simulink model "E55_1030"  (R2019b)
settings: Solver=FixedStepDiscrete  StartTime=0.0  StopTime=10  FixedStep=0.0005  RelTol=1e-3  EnableMultiTasking=on
InitFcn:
  | ecucoder_canfd
  | load('DATA_Plimit.mat')
  | a=0.775;
  | b=0.775;
  | kf=-50000;
  | kr=-50000;
  | m=226+75;
  | Iz=100;
  | u=0.85;
  | g=9.8;
  | L=a+b;
  | xi=0.1;
  | r=0.226;
  | Lw=1.171;
  | Tm=21;
  | i=15.9;
  | Jw=0.504;
  | Pmax=20000;
  | mw=19.3;
  | mb=148.9+75;
  | hg=0.280;
model workspace (MAT data in the model file):
  Initial_Steer_Position = 0
values from neighbouring files (symbols this model uses):
  SOC = [2.5 5 7.5 10 20 30 40 50 60 70 80 90 ... (14 elements, 14x1)]    [DATA_Plimit.mat]
  SOC_Discharge = [2.04592350211 2.57821618825 3.10671863859 3.63118835861 4.15200192786 4.66837694959 5.18149950051 5.69046162564 6.19532286188 6.696400261 7.19347596839 7.68712157998 ... (473 elements, 1x473)]    [DATA_Plimit.mat]
  VOLTAGE = [459.1488 476.0844 485.9448 487.344 492.822 498.8016 503.382 509.1108 518.8128 531.2472 544.5132 558.4656 ... (14 elements, 14x1)]    [DATA_Plimit.mat]
undefined symbols (not defined in the file or in its folder): DiscIntNeverNeededParam, H, HALL10, HALL6, HALL7, HALL8, HALL9, HPWM1, HPWM3, I_AN05_5V, I_AN07_5V, I_AN08_5V, I_AN09_5V, I_AN10_5V, I_SW11_H, I_SW12_H, I_SW13_H, I_SW14_H, I_SW15_H, I_SW16_H, I_SW17_H, I_SW18_H, I_SW19_H, LS1A2, O_HS1A2, O_HS1A8
libraries: ec311lib x152, simulink x92, canmsglib x30, canfdmsglib x2
(part 5 of 6)

== system E55_1030/Function-Call Subsystem2/Triggered Subsystem/AMK_Setpoints_Motor1 ==
  AMK_TorqueLimitNegativ_in : Inport
  AMK_TorqueLimitPositiv_in : Inport  Port=2
  AMK_TargetVelocity_in : Inport  Port=3
  AMK_Control_in : Inport  Port=4
  AMK_Control : Subsystem
  AMK_Setpoints_Motor1_DLC : Constant  Value=8  OutDataTypeStr=uint8
  AMK_Setpoints_Motor1_DLC_Out : Terminator
  AMK_Setpoints_Motor1_ID : Constant  Value=388  OutDataTypeStr=single
  AMK_Setpoints_Motor1_ID_Out : Terminator
  AMK_Setpoints_Motor1_mux : Mux  Inputs=8
  AMK_TargetVelocity : Subsystem
  AMK_TorqueLimitNegativ : Subsystem
  AMK_TorqueLimitPositiv : Subsystem
  Conv{1..8} (8 alike) : DataTypeConversion
  or{1..8} (8 alike) : simulink/Logic and Bit Operations/Bitwise Operator  logicop=OR  UseBitMask=off  NumInputPorts=4  BitMask=bin2dec('11011001')  BitMaskRealWorld=Stored Integer
  output : Outport
  wires:
  AMK_Setpoints_Motor1_mux/1 -> output/1
  AMK_TorqueLimitNegativ/1(output1) -> or1/1
  AMK_TorqueLimitNegativ/2(output2) -> or2/1
  AMK_TorqueLimitNegativ/3(output3) -> or3/1
  AMK_TorqueLimitNegativ/4(output4) -> or4/1
  AMK_TorqueLimitNegativ/5(output5) -> or5/1
  AMK_TorqueLimitNegativ/6(output6) -> or6/1
  AMK_TorqueLimitNegativ/7(output7) -> or7/1
  AMK_TorqueLimitNegativ/8(output8) -> or8/1
  AMK_TorqueLimitPositiv/1(output1) -> or1/2
  AMK_TorqueLimitPositiv/2(output2) -> or2/2
  AMK_TorqueLimitPositiv/3(output3) -> or3/2
  AMK_TorqueLimitPositiv/4(output4) -> or4/2
  AMK_TorqueLimitPositiv/5(output5) -> or5/2
  AMK_TorqueLimitPositiv/6(output6) -> or6/2
  AMK_TorqueLimitPositiv/7(output7) -> or7/2
  AMK_TorqueLimitPositiv/8(output8) -> or8/2
  AMK_TargetVelocity/1(output1) -> or1/3
  AMK_TargetVelocity/2(output2) -> or2/3
  AMK_TargetVelocity/3(output3) -> or3/3
  AMK_TargetVelocity/4(output4) -> or4/3
  AMK_TargetVelocity/5(output5) -> or5/3
  AMK_TargetVelocity/6(output6) -> or6/3
  AMK_TargetVelocity/7(output7) -> or7/3
  AMK_TargetVelocity/8(output8) -> or8/3
  AMK_Control/1(output1) -> or1/4
  AMK_Control/2(output2) -> or2/4
  AMK_Control/3(output3) -> or3/4
  AMK_Control/4(output4) -> or4/4
  AMK_Control/5(output5) -> or5/4
  AMK_Control/6(output6) -> or6/4
  AMK_Control/7(output7) -> or7/4
  AMK_Control/8(output8) -> or8/4
  or1/1 -> Conv1/1
  Conv1/1 -> AMK_Setpoints_Motor1_mux/1
  or2/1 -> Conv2/1
  Conv2/1 -> AMK_Setpoints_Motor1_mux/2
  or3/1 -> Conv3/1
  Conv3/1 -> AMK_Setpoints_Motor1_mux/3
  or4/1 -> Conv4/1
  Conv4/1 -> AMK_Setpoints_Motor1_mux/4
  or5/1 -> Conv5/1
  Conv5/1 -> AMK_Setpoints_Motor1_mux/5
  or6/1 -> Conv6/1
  Conv6/1 -> AMK_Setpoints_Motor1_mux/6
  or7/1 -> Conv7/1
  Conv7/1 -> AMK_Setpoints_Motor1_mux/7
  or8/1 -> Conv8/1
  Conv8/1 -> AMK_Setpoints_Motor1_mux/8
  AMK_Setpoints_Motor1_ID/1 -> AMK_Setpoints_Motor1_ID_Out/1
  AMK_Setpoints_Motor1_DLC/1 -> AMK_Setpoints_Motor1_DLC_Out/1
  AMK_TorqueLimitNegativ_in/1 -> AMK_TorqueLimitNegativ/1(AMK_TorqueLimitNegativ)
  AMK_TorqueLimitPositiv_in/1 -> AMK_TorqueLimitPositiv/1(AMK_TorqueLimitPositiv)
  AMK_TargetVelocity_in/1 -> AMK_TargetVelocity/1(AMK_TargetVelocity)
  AMK_Control_in/1 -> AMK_Control/1(AMK_Control)

== system E55_1030/Function-Call Subsystem2/Triggered Subsystem/AMK_Setpoints_Motor2 ==
  AMK_TorqueLimitNegativ_in : Inport
  AMK_TorqueLimitPositiv_in : Inport  Port=2
  AMK_TargetVelocity_in : Inport  Port=3
  AMK_Control_in : Inport  Port=4
  AMK_Control : Subsystem
  AMK_Setpoints_Motor1_DLC : Constant  Value=8  OutDataTypeStr=uint8
  AMK_Setpoints_Motor1_DLC_Out : Terminator
  AMK_Setpoints_Motor1_ID : Constant  Value=388  OutDataTypeStr=single
  AMK_Setpoints_Motor1_ID_Out : Terminator
  AMK_Setpoints_Motor1_mux : Mux  Inputs=8
  AMK_TargetVelocity : Subsystem
  AMK_TorqueLimitNegativ : Subsystem
  AMK_TorqueLimitPositiv : Subsystem
  Conv{1..8} (8 alike) : DataTypeConversion
  or{1..8} (8 alike) : simulink/Logic and Bit Operations/Bitwise Operator  logicop=OR  UseBitMask=off  NumInputPorts=4  BitMask=bin2dec('11011001')  BitMaskRealWorld=Stored Integer
  output : Outport
  wires:
  AMK_Control_in/1 -> AMK_Control/1(AMK_Control)
  AMK_TargetVelocity_in/1 -> AMK_TargetVelocity/1(AMK_TargetVelocity)
  AMK_TorqueLimitPositiv_in/1 -> AMK_TorqueLimitPositiv/1(AMK_TorqueLimitPositiv)
  AMK_TorqueLimitNegativ_in/1 -> AMK_TorqueLimitNegativ/1(AMK_TorqueLimitNegativ)
  AMK_Setpoints_Motor1_DLC/1 -> AMK_Setpoints_Motor1_DLC_Out/1
  AMK_Setpoints_Motor1_ID/1 -> AMK_Setpoints_Motor1_ID_Out/1
  Conv8/1 -> AMK_Setpoints_Motor1_mux/8
  or8/1 -> Conv8/1
  Conv7/1 -> AMK_Setpoints_Motor1_mux/7
  or7/1 -> Conv7/1
  Conv6/1 -> AMK_Setpoints_Motor1_mux/6
  or6/1 -> Conv6/1
  Conv5/1 -> AMK_Setpoints_Motor1_mux/5
  or5/1 -> Conv5/1
  Conv4/1 -> AMK_Setpoints_Motor1_mux/4
  or4/1 -> Conv4/1
  Conv3/1 -> AMK_Setpoints_Motor1_mux/3
  or3/1 -> Conv3/1
  Conv2/1 -> AMK_Setpoints_Motor1_mux/2
  or2/1 -> Conv2/1
  Conv1/1 -> AMK_Setpoints_Motor1_mux/1
  or1/1 -> Conv1/1
  AMK_Control/8(output8) -> or8/4
  AMK_Control/7(output7) -> or7/4
  AMK_Control/6(output6) -> or6/4
  AMK_Control/5(output5) -> or5/4
  AMK_Control/4(output4) -> or4/4
  AMK_Control/3(output3) -> or3/4
  AMK_Control/2(output2) -> or2/4
  AMK_Control/1(output1) -> or1/4
  AMK_TargetVelocity/8(output8) -> or8/3
  AMK_TargetVelocity/7(output7) -> or7/3
  AMK_TargetVelocity/6(output6) -> or6/3
  AMK_TargetVelocity/5(output5) -> or5/3
  AMK_TargetVelocity/4(output4) -> or4/3
  AMK_TargetVelocity/3(output3) -> or3/3
  AMK_TargetVelocity/2(output2) -> or2/3
  AMK_TargetVelocity/1(output1) -> or1/3
  AMK_TorqueLimitPositiv/8(output8) -> or8/2
  AMK_TorqueLimitPositiv/7(output7) -> or7/2
  AMK_TorqueLimitPositiv/6(output6) -> or6/2
  AMK_TorqueLimitPositiv/5(output5) -> or5/2
  AMK_TorqueLimitPositiv/4(output4) -> or4/2
  AMK_TorqueLimitPositiv/3(output3) -> or3/2
  AMK_TorqueLimitPositiv/2(output2) -> or2/2
  AMK_TorqueLimitPositiv/1(output1) -> or1/2
  AMK_TorqueLimitNegativ/8(output8) -> or8/1
  AMK_TorqueLimitNegativ/7(output7) -> or7/1
  AMK_TorqueLimitNegativ/6(output6) -> or6/1
  AMK_TorqueLimitNegativ/5(output5) -> or5/1
  AMK_TorqueLimitNegativ/4(output4) -> or4/1
  AMK_TorqueLimitNegativ/3(output3) -> or3/1
  AMK_TorqueLimitNegativ/2(output2) -> or2/1
  AMK_TorqueLimitNegativ/1(output1) -> or1/1
  AMK_Setpoints_Motor1_mux/1 -> output/1

== system E55_1030/Function-Call Subsystem2/Triggered Subsystem/AMK_Setpoints_Motor3 ==
  AMK_TorqueLimitNegativ_in : Inport
  AMK_TorqueLimitPositiv_in : Inport  Port=2
  AMK_TargetVelocity_in : Inport  Port=3
  AMK_Control_in : Inport  Port=4
  AMK_Control : Subsystem
  AMK_Setpoints_Motor1_DLC : Constant  Value=8  OutDataTypeStr=uint8
  AMK_Setpoints_Motor1_DLC_Out : Terminator
  AMK_Setpoints_Motor1_ID : Constant  Value=388  OutDataTypeStr=single
  AMK_Setpoints_Motor1_ID_Out : Terminator
  AMK_Setpoints_Motor1_mux : Mux  Inputs=8
  AMK_TargetVelocity : Subsystem
  AMK_TorqueLimitNegativ : Subsystem
  AMK_TorqueLimitPositiv : Subsystem
  Conv{1..8} (8 alike) : DataTypeConversion
  or{1..8} (8 alike) : simulink/Logic and Bit Operations/Bitwise Operator  logicop=OR  UseBitMask=off  NumInputPorts=4  BitMask=bin2dec('11011001')  BitMaskRealWorld=Stored Integer
  output : Outport
  wires:
  AMK_Control_in/1 -> AMK_Control/1(AMK_Control)
  AMK_TargetVelocity_in/1 -> AMK_TargetVelocity/1(AMK_TargetVelocity)
  AMK_TorqueLimitPositiv_in/1 -> AMK_TorqueLimitPositiv/1(AMK_TorqueLimitPositiv)
  AMK_TorqueLimitNegativ_in/1 -> AMK_TorqueLimitNegativ/1(AMK_TorqueLimitNegativ)
  AMK_Setpoints_Motor1_DLC/1 -> AMK_Setpoints_Motor1_DLC_Out/1
  AMK_Setpoints_Motor1_ID/1 -> AMK_Setpoints_Motor1_ID_Out/1
  Conv8/1 -> AMK_Setpoints_Motor1_mux/8
  or8/1 -> Conv8/1
  Conv7/1 -> AMK_Setpoints_Motor1_mux/7
  or7/1 -> Conv7/1
  Conv6/1 -> AMK_Setpoints_Motor1_mux/6
  or6/1 -> Conv6/1
  Conv5/1 -> AMK_Setpoints_Motor1_mux/5
  or5/1 -> Conv5/1
  Conv4/1 -> AMK_Setpoints_Motor1_mux/4
  or4/1 -> Conv4/1
  Conv3/1 -> AMK_Setpoints_Motor1_mux/3
  or3/1 -> Conv3/1
  Conv2/1 -> AMK_Setpoints_Motor1_mux/2
  or2/1 -> Conv2/1
  Conv1/1 -> AMK_Setpoints_Motor1_mux/1
  or1/1 -> Conv1/1
  AMK_Control/8(output8) -> or8/4
  AMK_Control/7(output7) -> or7/4
  AMK_Control/6(output6) -> or6/4
  AMK_Control/5(output5) -> or5/4
  AMK_Control/4(output4) -> or4/4
  AMK_Control/3(output3) -> or3/4
  AMK_Control/2(output2) -> or2/4
  AMK_Control/1(output1) -> or1/4
  AMK_TargetVelocity/8(output8) -> or8/3
  AMK_TargetVelocity/7(output7) -> or7/3
  AMK_TargetVelocity/6(output6) -> or6/3
  AMK_TargetVelocity/5(output5) -> or5/3
  AMK_TargetVelocity/4(output4) -> or4/3
  AMK_TargetVelocity/3(output3) -> or3/3
  AMK_TargetVelocity/2(output2) -> or2/3
  AMK_TargetVelocity/1(output1) -> or1/3
  AMK_TorqueLimitPositiv/8(output8) -> or8/2
  AMK_TorqueLimitPositiv/7(output7) -> or7/2
  AMK_TorqueLimitPositiv/6(output6) -> or6/2
  AMK_TorqueLimitPositiv/5(output5) -> or5/2
  AMK_TorqueLimitPositiv/4(output4) -> or4/2
  AMK_TorqueLimitPositiv/3(output3) -> or3/2
  AMK_TorqueLimitPositiv/2(output2) -> or2/2
  AMK_TorqueLimitPositiv/1(output1) -> or1/2
  AMK_TorqueLimitNegativ/8(output8) -> or8/1
  AMK_TorqueLimitNegativ/7(output7) -> or7/1
  AMK_TorqueLimitNegativ/6(output6) -> or6/1
  AMK_TorqueLimitNegativ/5(output5) -> or5/1
  AMK_TorqueLimitNegativ/4(output4) -> or4/1
  AMK_TorqueLimitNegativ/3(output3) -> or3/1
  AMK_TorqueLimitNegativ/2(output2) -> or2/1
  AMK_TorqueLimitNegativ/1(output1) -> or1/1
  AMK_Setpoints_Motor1_mux/1 -> output/1

== system E55_1030/Function-Call Subsystem2/Triggered Subsystem/AMK_Setpoints_Motor4 ==
  AMK_TorqueLimitNegativ_in : Inport
  AMK_TorqueLimitPositiv_in : Inport  Port=2
  AMK_TargetVelocity_in : Inport  Port=3
  AMK_Control_in : Inport  Port=4
  AMK_Control : Subsystem
  AMK_Setpoints_Motor1_DLC : Constant  Value=8  OutDataTypeStr=uint8
  AMK_Setpoints_Motor1_DLC_Out : Terminator
  AMK_Setpoints_Motor1_ID : Constant  Value=388  OutDataTypeStr=single
  AMK_Setpoints_Motor1_ID_Out : Terminator
  AMK_Setpoints_Motor1_mux : Mux  Inputs=8
  AMK_TargetVelocity : Subsystem
  AMK_TorqueLimitNegativ : Subsystem
  AMK_TorqueLimitPositiv : Subsystem
  Conv{1..8} (8 alike) : DataTypeConversion
  or{1..8} (8 alike) : simulink/Logic and Bit Operations/Bitwise Operator  logicop=OR  UseBitMask=off  NumInputPorts=4  BitMask=bin2dec('11011001')  BitMaskRealWorld=Stored Integer
  output : Outport
  wires:
  AMK_Setpoints_Motor1_mux/1 -> output/1
  AMK_TorqueLimitNegativ/1(output1) -> or1/1
  AMK_TorqueLimitNegativ/2(output2) -> or2/1
  AMK_TorqueLimitNegativ/3(output3) -> or3/1
  AMK_TorqueLimitNegativ/4(output4) -> or4/1
  AMK_TorqueLimitNegativ/5(output5) -> or5/1
  AMK_TorqueLimitNegativ/6(output6) -> or6/1
  AMK_TorqueLimitNegativ/7(output7) -> or7/1
  AMK_TorqueLimitNegativ/8(output8) -> or8/1
  AMK_TorqueLimitPositiv/1(output1) -> or1/2
  AMK_TorqueLimitPositiv/2(output2) -> or2/2
  AMK_TorqueLimitPositiv/3(output3) -> or3/2
  AMK_TorqueLimitPositiv/4(output4) -> or4/2
  AMK_TorqueLimitPositiv/5(output5) -> or5/2
  AMK_TorqueLimitPositiv/6(output6) -> or6/2
  AMK_TorqueLimitPositiv/7(output7) -> or7/2
  AMK_TorqueLimitPositiv/8(output8) -> or8/2
  AMK_TargetVelocity/1(output1) -> or1/3
  AMK_TargetVelocity/2(output2) -> or2/3
  AMK_TargetVelocity/3(output3) -> or3/3
  AMK_TargetVelocity/4(output4) -> or4/3
  AMK_TargetVelocity/5(output5) -> or5/3
  AMK_TargetVelocity/6(output6) -> or6/3
  AMK_TargetVelocity/7(output7) -> or7/3
  AMK_TargetVelocity/8(output8) -> or8/3
  AMK_Control/1(output1) -> or1/4
  AMK_Control/2(output2) -> or2/4
  AMK_Control/3(output3) -> or3/4
  AMK_Control/4(output4) -> or4/4
  AMK_Control/5(output5) -> or5/4
  AMK_Control/6(output6) -> or6/4
  AMK_Control/7(output7) -> or7/4
  AMK_Control/8(output8) -> or8/4
  or1/1 -> Conv1/1
  Conv1/1 -> AMK_Setpoints_Motor1_mux/1
  or2/1 -> Conv2/1
  Conv2/1 -> AMK_Setpoints_Motor1_mux/2
  or3/1 -> Conv3/1
  Conv3/1 -> AMK_Setpoints_Motor1_mux/3
  or4/1 -> Conv4/1
  Conv4/1 -> AMK_Setpoints_Motor1_mux/4
  or5/1 -> Conv5/1
  Conv5/1 -> AMK_Setpoints_Motor1_mux/5
  or6/1 -> Conv6/1
  Conv6/1 -> AMK_Setpoints_Motor1_mux/6
  or7/1 -> Conv7/1
  Conv7/1 -> AMK_Setpoints_Motor1_mux/7
  or8/1 -> Conv8/1
  Conv8/1 -> AMK_Setpoints_Motor1_mux/8
  AMK_Setpoints_Motor1_ID/1 -> AMK_Setpoints_Motor1_ID_Out/1
  AMK_Setpoints_Motor1_DLC/1 -> AMK_Setpoints_Motor1_DLC_Out/1
  AMK_TorqueLimitNegativ_in/1 -> AMK_TorqueLimitNegativ/1(AMK_TorqueLimitNegativ)
  AMK_TorqueLimitPositiv_in/1 -> AMK_TorqueLimitPositiv/1(AMK_TorqueLimitPositiv)
  AMK_TargetVelocity_in/1 -> AMK_TargetVelocity/1(AMK_TargetVelocity)
  AMK_Control_in/1 -> AMK_Control/1(AMK_Control)

== system E55_1030/Function-Call Subsystem2/计算理想横摆角速度和质心侧偏角/线性二自由度模型 ==
  steer_angle_rad : Inport
  velocity_m/s : Inport  Port=2
  Add : Sum  Inputs=++-
  Add1 : Sum  Inputs=+-
  Add2 : Sum  Inputs=++-
  Discrete-Time Integrator : DiscreteIntegrator  SampleTime=-1  ICPrevOutput=DiscIntNeverNeededParam  ICPrevScaledInput=DiscIntNeverNeededParam
  Discrete-Time Integrator1 : DiscreteIntegrator  SampleTime=-1  ICPrevOutput=DiscIntNeverNeededParam  ICPrevScaledInput=DiscIntNeverNeededParam
  Divide{,1..2,4} (4 alike) : Product  Inputs=*/
  Divide3 : Product  Inputs=**
  Gain2 : Gain  Gain=kf+kr
  Gain3 : Gain  Gain=a*kf-b*kr
  Gain4 : Gain  Gain=kf
  Gain5 : Gain  Gain=a*kf-b*kr
  Gain6 : Gain  Gain=a^2*kf+b^2*kr
  Gain7 : Gain  Gain=a*kr
  Gain8 : Gain  Gain=180/pi
  Gain9 : Gain  Gain=180/pi
  Iz_kg*m^2 : Constant  Value=Iz
  m_kg : Constant  Value=m
  side_slip_angle_° : Outport
  yaw_rate_°/s : Outport  Port=2
  wires:
  steer_angle_rad/1 -> Gain7/1, Gain4/1
  Gain3/1 -> Add/2
  velocity_m/s/1 -> Divide1/2, Divide3/2, Divide/2
  m_kg/1 -> Divide2/2
  Divide1/1 -> Gain3/1, Gain6/1
  Gain7/1 -> Add2/3
  Discrete-Time Integrator1/1 -> Gain9/1, Divide3/1, Divide1/1
  Divide2/1 -> Add1/1
  Divide/1 -> Gain8/1, Gain2/1, Gain5/1
  Gain6/1 -> Add2/2
  Add1/1 -> Discrete-Time Integrator/1
  Divide3/1 -> Add1/2
  Add2/1 -> Divide4/1
  Add/1 -> Divide2/1
  Gain4/1 -> Add/3
  Gain5/1 -> Add2/1
  Divide4/1 -> Discrete-Time Integrator1/1
  Gain2/1 -> Add/1
  Iz_kg*m^2/1 -> Divide4/2
  Discrete-Time Integrator/1 -> Divide/1
  Gain8/1 -> side_slip_angle_°/1
  Gain9/1 -> yaw_rate_°/s/1

== system E55_1030/Function-Call Subsystem2/计算理想转速/计算右前理想转速 ==
  velocity : Inport
  Yaw_Rate : Inport  Port=2
  steer_angle : Inport  Port=3
  Abs2 : Abs
  Add1 : Sum
  Constant3 : Constant  Value=r
  Cos : Trigonometry  Operator=cos
  Divide1 : Product  Inputs=**/
  Gain6 : Gain  Gain=Lw/2
  wheel_speed_d_fr : Outport
  wires:
  Divide1/1 -> wheel_speed_d_fr/1
  Add1/1 -> Divide1/1
  Abs2/1 -> Divide1/2
  steer_angle/1 -> Cos/1
  Cos/1 -> Abs2/1
  Constant3/1 -> Divide1/3
  Gain6/1 -> Add1/2
  velocity/1 -> Add1/1
  Yaw_Rate/1 -> Gain6/1

== system E55_1030/Function-Call Subsystem2/计算理想转速/计算右后理想转速 ==
  velocity : Inport
  Yaw_Rate : Inport  Port=2
  Add1 : Sum
  Constant3 : Constant  Value=r
  Divide1 : Product  Inputs=*/
  Gain6 : Gain  Gain=Lw/2
  wheel_speed_d_rr : Outport
  wires:
  Yaw_Rate/1 -> Gain6/1
  velocity/1 -> Add1/1
  Gain6/1 -> Add1/2
  Constant3/1 -> Divide1/2
  Add1/1 -> Divide1/1
  Divide1/1 -> wheel_speed_d_rr/1

== system E55_1030/Function-Call Subsystem2/计算理想转速/计算左前理想转速 ==
  velocity : Inport
  Yaw_Rate : Inport  Port=2
  steer_angle : Inport  Port=3
  Abs2 : Abs
  Add1 : Sum  Inputs=+-
  Constant3 : Constant  Value=r
  Cos : Trigonometry  Operator=cos
  Divide1 : Product  Inputs=**/
  Gain6 : Gain  Gain=Lw/2
  wheel_speed_d_fl : Outport
  wires:
  Yaw_Rate/1 -> Gain6/1
  velocity/1 -> Add1/1
  Gain6/1 -> Add1/2
  Constant3/1 -> Divide1/3
  Cos/1 -> Abs2/1
  steer_angle/1 -> Cos/1
  Abs2/1 -> Divide1/2
  Add1/1 -> Divide1/1
  Divide1/1 -> wheel_speed_d_fl/1

== system E55_1030/Function-Call Subsystem2/计算理想转速/计算左后理想转速 ==
  velocity : Inport
  Yaw_Rate : Inport  Port=2
  Add1 : Sum  Inputs=+-
  Constant3 : Constant  Value=r
  Divide1 : Product  Inputs=*/
  Gain6 : Gain  Gain=Lw/2
  wheel_speed_d_rl : Outport
  wires:
  Divide1/1 -> wheel_speed_d_rl/1
  Add1/1 -> Divide1/1
  Constant3/1 -> Divide1/2
  Gain6/1 -> Add1/2
  velocity/1 -> Add1/1
  Yaw_Rate/1 -> Gain6/1

== system E55_1030/Function-Call Subsystem2/Triggered Subsystem/AMK_Setpoints_Motor1/AMK_Control ==
  AMK_Control : Inport
  AMK_ControlCOV : DataTypeConversion  OutDataTypeStr=uint8
  AMK_ControlRon : Rounding  Operator=round
  AMK_Control_1sat : Saturate  UpperLimit=65535  LowerLimit=0
  AMK_Control_And : simulink/Logic and Bit Operations/Bitwise Operator  logicop=AND  UseBitMask=off  NumInputPorts=2  BitMask=bin2dec('11011001')  BitMaskRealWorld=Stored Integer
  AMK_Control_And_C : Constant  Value=255  OutDataTypeStr=uint32
  AMK_Control_Convert : DataTypeConversion  OutDataTypeStr=uint32
  AMK_Control_D : Product  Inputs=*/
  AMK_Control_D1 : Product  Inputs=*/
  AMK_Control_F : Constant  OutDataTypeStr=single
  AMK_Control_L : simulink/Logic and Bit Operations/Bitwise Operator  logicop=AND  UseBitMask=on  BitMask=65535  BitMaskRealWorld=Stored Integer
  AMK_Control_O : Constant  Value=0  OutDataTypeStr=single
  AMK_Control_S : ArithShift
  AMK_Control_sat : Saturate  UpperLimit=65535  LowerLimit=0
  AMK_Control_st : Sum  Inputs=+-
  AMK_Controloutput2_C : Constant  Value=256
  BitCov : DataTypeConversion  OutDataTypeStr=uint8
  Constant{3..8} (6 alike) : Constant  Value=0  OutDataTypeStr=uint8  SampleTime=-1
  output1 : Outport
  output2 : Outport  Port=2
  output3 : Outport  Port=3
  output4 : Outport  Port=4
  output5 : Outport  Port=5
  output6 : Outport  Port=6
  output7 : Outport  Port=7
  output8 : Outport  Port=8
  wires:
  AMK_Control/1 -> AMK_Control_sat/1
  AMK_Control_sat/1 -> AMK_Control_st/1
  AMK_Control_O/1 -> AMK_Control_st/2
  AMK_Control_st/1 -> AMK_Control_D/1
  AMK_Control_F/1 -> AMK_Control_D/2
  AMK_Control_D/1 -> AMK_ControlRon/1
  AMK_ControlRon/1 -> AMK_Control_S/1
  AMK_Control_S/1 -> AMK_Control_1sat/1
  AMK_Control_1sat/1 -> AMK_Control_Convert/1
  AMK_Control_Convert/1 -> AMK_Control_L/1
  AMK_Control_L/1 -> AMK_Control_D1/1, AMK_Control_And/1
  AMK_Controloutput2_C/1 -> AMK_Control_D1/2
  AMK_Control_D1/1 -> AMK_ControlCOV/1
  AMK_ControlCOV/1 -> output2/1
  AMK_Control_And_C/1 -> AMK_Control_And/2
  AMK_Control_And/1 -> BitCov/1
  BitCov/1 -> output1/1
  Constant3/1 -> output3/1
  Constant4/1 -> output4/1
  Constant5/1 -> output5/1
  Constant6/1 -> output6/1
  Constant7/1 -> output7/1
  Constant8/1 -> output8/1

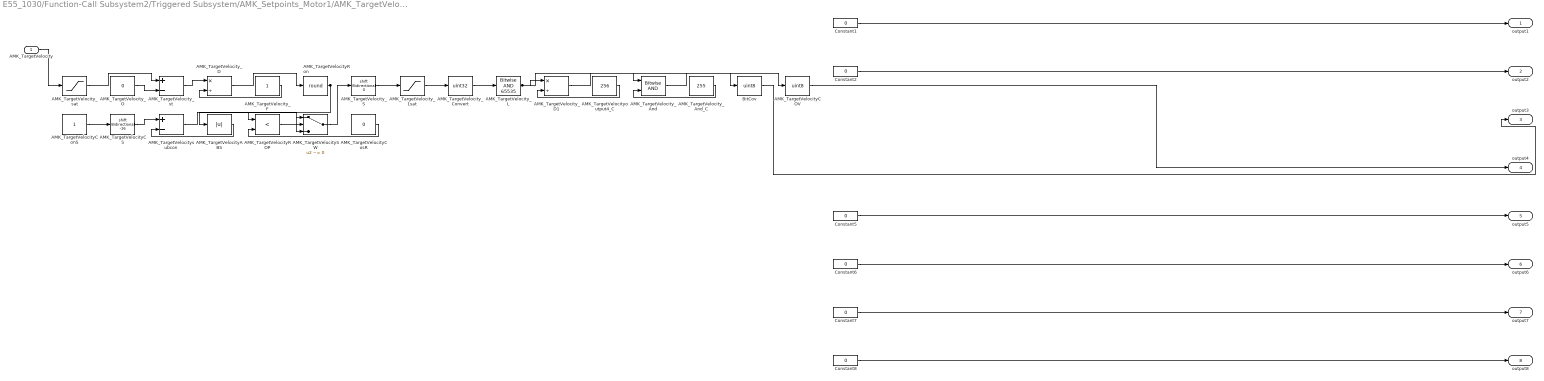
== system E55_1030/Function-Call Subsystem2/Triggered Subsystem/AMK_Setpoints_Motor1/AMK_TargetVelocity ==
  AMK_TargetVelocity : Inport
  AMK_TargetVelocityABS : Abs
  AMK_TargetVelocityCOV : DataTypeConversion  OutDataTypeStr=uint8
  AMK_TargetVelocityCS : ArithShift  BitShiftNumber=-16
  AMK_TargetVelocityConS : Constant  OutDataTypeStr=single
  AMK_TargetVelocityCosR : Constant  Value=0  OutDataTypeStr=uint8
  AMK_TargetVelocityROP : RelationalOperator  Operator=<  OutDataTypeStr=boolean  RndMeth=Nearest
  AMK_TargetVelocityRon : Rounding  Operator=round
  AMK_TargetVelocitySW : Switch  Criteria=u2 ~= 0
  AMK_TargetVelocity_1sat : Saturate  UpperLimit=65535  LowerLimit=0
  AMK_TargetVelocity_And : simulink/Logic and Bit Operations/Bitwise Operator  logicop=AND  UseBitMask=off  NumInputPorts=2  BitMask=bin2dec('11011001')  BitMaskRealWorld=Stored Integer
  AMK_TargetVelocity_And_C : Constant  Value=255  OutDataTypeStr=uint32
  AMK_TargetVelocity_Convert : DataTypeConversion  OutDataTypeStr=uint32
  AMK_TargetVelocity_D : Product  Inputs=*/
  AMK_TargetVelocity_D1 : Product  Inputs=*/
  AMK_TargetVelocity_F : Constant  OutDataTypeStr=single
  AMK_TargetVelocity_L : simulink/Logic and Bit Operations/Bitwise Operator  logicop=AND  UseBitMask=on  BitMask=65535  BitMaskRealWorld=Stored Integer
  AMK_TargetVelocity_O : Constant  Value=0  OutDataTypeStr=single
  AMK_TargetVelocity_S : ArithShift
  AMK_TargetVelocity_sat : Saturate  UpperLimit=32767  LowerLimit=-32768
  AMK_TargetVelocity_st : Sum  Inputs=+-
  AMK_TargetVelocityoutput4_C : Constant  Value=256
  AMK_TargetVelocitysubcon : Sum  Inputs=+-
  BitCov : DataTypeConversion  OutDataTypeStr=uint8
  Constant{1..2,5..8} (6 alike) : Constant  Value=0  OutDataTypeStr=uint8  SampleTime=-1
  output1 : Outport
  output2 : Outport  Port=2
  output3 : Outport  Port=3
  output4 : Outport  Port=4
  output5 : Outport  Port=5
  output6 : Outport  Port=6
  output7 : Outport  Port=7
  output8 : Outport  Port=8
  wires:
  AMK_TargetVelocity/1 -> AMK_TargetVelocity_sat/1
  AMK_TargetVelocity_sat/1 -> AMK_TargetVelocity_st/1
  AMK_TargetVelocity_O/1 -> AMK_TargetVelocity_st/2
  AMK_TargetVelocity_st/1 -> AMK_TargetVelocity_D/1
  AMK_TargetVelocity_F/1 -> AMK_TargetVelocity_D/2
  AMK_TargetVelocity_D/1 -> AMK_TargetVelocityRon/1
  AMK_TargetVelocityRon/1 -> AMK_TargetVelocityROP/1, AMK_TargetVelocityABS/1, AMK_TargetVelocitySW/3
  AMK_TargetVelocityCosR/1 -> AMK_TargetVelocityROP/2
  AMK_TargetVelocityConS/1 -> AMK_TargetVelocityCS/1
  AMK_TargetVelocityCS/1 -> AMK_TargetVelocitysubcon/1
  AMK_TargetVelocityABS/1 -> AMK_TargetVelocitysubcon/2
  AMK_TargetVelocitysubcon/1 -> AMK_TargetVelocitySW/1
  AMK_TargetVelocityROP/1 -> AMK_TargetVelocitySW/2
  AMK_TargetVelocitySW/1 -> AMK_TargetVelocity_S/1
  AMK_TargetVelocity_S/1 -> AMK_TargetVelocity_1sat/1
  AMK_TargetVelocity_1sat/1 -> AMK_TargetVelocity_Convert/1
  AMK_TargetVelocity_Convert/1 -> AMK_TargetVelocity_L/1
  AMK_TargetVelocity_L/1 -> AMK_TargetVelocity_D1/1, AMK_TargetVelocity_And/1
  AMK_TargetVelocityoutput4_C/1 -> AMK_TargetVelocity_D1/2
  AMK_TargetVelocity_D1/1 -> AMK_TargetVelocityCOV/1
  AMK_TargetVelocityCOV/1 -> output4/1
  AMK_TargetVelocity_And_C/1 -> AMK_TargetVelocity_And/2
  AMK_TargetVelocity_And/1 -> BitCov/1
  BitCov/1 -> output3/1
  Constant1/1 -> output1/1
  Constant2/1 -> output2/1
  Constant5/1 -> output5/1
  Constant6/1 -> output6/1
  Constant7/1 -> output7/1
  Constant8/1 -> output8/1

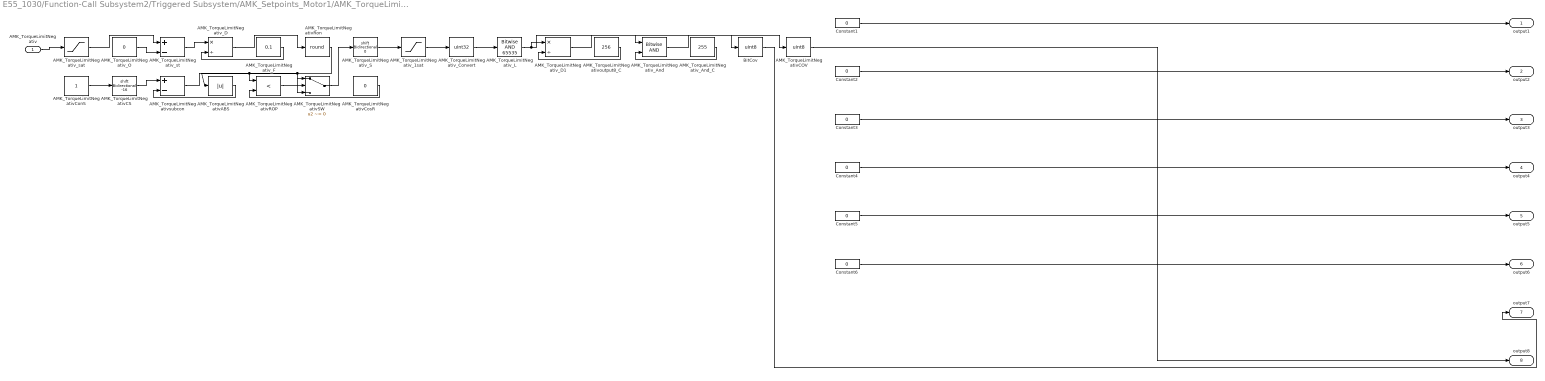
== system E55_1030/Function-Call Subsystem2/Triggered Subsystem/AMK_Setpoints_Motor1/AMK_TorqueLimitNegativ ==
  AMK_TorqueLimitNegativ : Inport
  AMK_TorqueLimitNegativABS : Abs
  AMK_TorqueLimitNegativCOV : DataTypeConversion  OutDataTypeStr=uint8
  AMK_TorqueLimitNegativCS : ArithShift  BitShiftNumber=-16
  AMK_TorqueLimitNegativConS : Constant  OutDataTypeStr=single
  AMK_TorqueLimitNegativCosR : Constant  Value=0  OutDataTypeStr=uint8
  AMK_TorqueLimitNegativROP : RelationalOperator  Operator=<  OutDataTypeStr=boolean  RndMeth=Nearest
  AMK_TorqueLimitNegativRon : Rounding  Operator=round
  AMK_TorqueLimitNegativSW : Switch  Criteria=u2 ~= 0
  AMK_TorqueLimitNegativ_1sat : Saturate  UpperLimit=65535  LowerLimit=0
  AMK_TorqueLimitNegativ_And : simulink/Logic and Bit Operations/Bitwise Operator  logicop=AND  UseBitMask=off  NumInputPorts=2  BitMask=bin2dec('11011001')  BitMaskRealWorld=Stored Integer
  AMK_TorqueLimitNegativ_And_C : Constant  Value=255  OutDataTypeStr=uint32
  AMK_TorqueLimitNegativ_Convert : DataTypeConversion  OutDataTypeStr=uint32
  AMK_TorqueLimitNegativ_D : Product  Inputs=*/
  AMK_TorqueLimitNegativ_D1 : Product  Inputs=*/
  AMK_TorqueLimitNegativ_F : Constant  Value=0.1  OutDataTypeStr=single
  AMK_TorqueLimitNegativ_L : simulink/Logic and Bit Operations/Bitwise Operator  logicop=AND  UseBitMask=on  BitMask=65535  BitMaskRealWorld=Stored Integer
  AMK_TorqueLimitNegativ_O : Constant  Value=0  OutDataTypeStr=single
  AMK_TorqueLimitNegativ_S : ArithShift
  AMK_TorqueLimitNegativ_sat : Saturate  UpperLimit=0  LowerLimit=-100
  AMK_TorqueLimitNegativ_st : Sum  Inputs=+-
  AMK_TorqueLimitNegativoutput8_C : Constant  Value=256
  AMK_TorqueLimitNegativsubcon : Sum  Inputs=+-
  BitCov : DataTypeConversion  OutDataTypeStr=uint8
  Constant{1..6} (6 alike) : Constant  Value=0  OutDataTypeStr=uint8  SampleTime=-1
  output1 : Outport
  output2 : Outport  Port=2
  output3 : Outport  Port=3
  output4 : Outport  Port=4
  output5 : Outport  Port=5
  output6 : Outport  Port=6
  output7 : Outport  Port=7
  output8 : Outport  Port=8
  wires:
  AMK_TorqueLimitNegativ/1 -> AMK_TorqueLimitNegativ_sat/1
  AMK_TorqueLimitNegativ_sat/1 -> AMK_TorqueLimitNegativ_st/1
  AMK_TorqueLimitNegativ_O/1 -> AMK_TorqueLimitNegativ_st/2
  AMK_TorqueLimitNegativ_st/1 -> AMK_TorqueLimitNegativ_D/1
  AMK_TorqueLimitNegativ_F/1 -> AMK_TorqueLimitNegativ_D/2
  AMK_TorqueLimitNegativ_D/1 -> AMK_TorqueLimitNegativRon/1
  AMK_TorqueLimitNegativRon/1 -> AMK_TorqueLimitNegativROP/1, AMK_TorqueLimitNegativABS/1, AMK_TorqueLimitNegativSW/3
  AMK_TorqueLimitNegativCosR/1 -> AMK_TorqueLimitNegativROP/2
  AMK_TorqueLimitNegativConS/1 -> AMK_TorqueLimitNegativCS/1
  AMK_TorqueLimitNegativCS/1 -> AMK_TorqueLimitNegativsubcon/1
  AMK_TorqueLimitNegativABS/1 -> AMK_TorqueLimitNegativsubcon/2
  AMK_TorqueLimitNegativsubcon/1 -> AMK_TorqueLimitNegativSW/1
  AMK_TorqueLimitNegativROP/1 -> AMK_TorqueLimitNegativSW/2
  AMK_TorqueLimitNegativSW/1 -> AMK_TorqueLimitNegativ_S/1
  AMK_TorqueLimitNegativ_S/1 -> AMK_TorqueLimitNegativ_1sat/1
  AMK_TorqueLimitNegativ_1sat/1 -> AMK_TorqueLimitNegativ_Convert/1
  AMK_TorqueLimitNegativ_Convert/1 -> AMK_TorqueLimitNegativ_L/1
  AMK_TorqueLimitNegativ_L/1 -> AMK_TorqueLimitNegativ_D1/1, AMK_TorqueLimitNegativ_And/1
  AMK_TorqueLimitNegativoutput8_C/1 -> AMK_TorqueLimitNegativ_D1/2
  AMK_TorqueLimitNegativ_D1/1 -> AMK_TorqueLimitNegativCOV/1
  AMK_TorqueLimitNegativCOV/1 -> output8/1
  AMK_TorqueLimitNegativ_And_C/1 -> AMK_TorqueLimitNegativ_And/2
  AMK_TorqueLimitNegativ_And/1 -> BitCov/1
  BitCov/1 -> output7/1
  Constant1/1 -> output1/1
  Constant2/1 -> output2/1
  Constant3/1 -> output3/1
  Constant4/1 -> output4/1
  Constant5/1 -> output5/1
  Constant6/1 -> output6/1

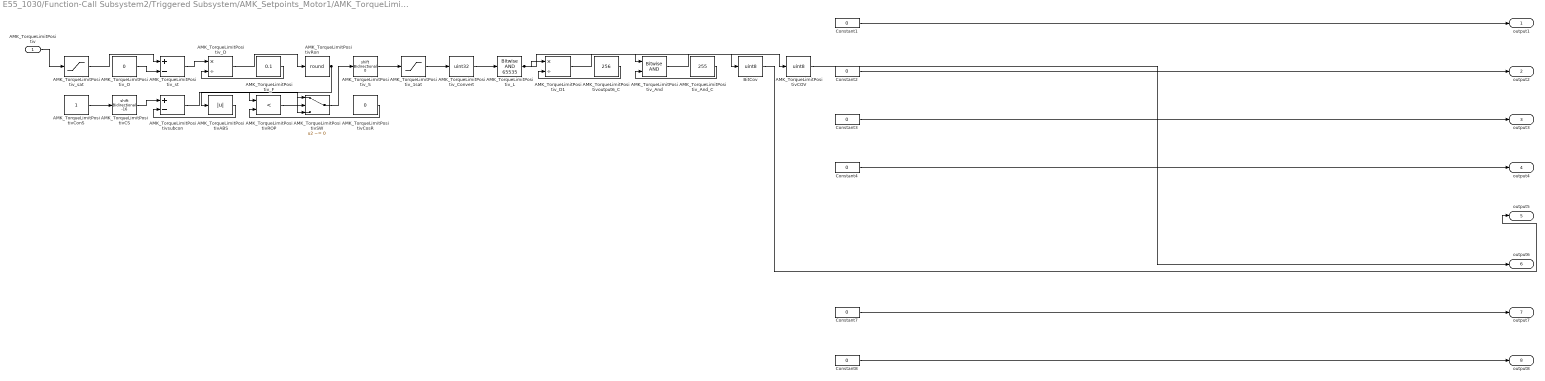
== system E55_1030/Function-Call Subsystem2/Triggered Subsystem/AMK_Setpoints_Motor1/AMK_TorqueLimitPositiv ==
  AMK_TorqueLimitPositiv : Inport
  AMK_TorqueLimitPositivABS : Abs
  AMK_TorqueLimitPositivCOV : DataTypeConversion  OutDataTypeStr=uint8
  AMK_TorqueLimitPositivCS : ArithShift  BitShiftNumber=-16
  AMK_TorqueLimitPositivConS : Constant  OutDataTypeStr=single
  AMK_TorqueLimitPositivCosR : Constant  Value=0  OutDataTypeStr=uint8
  AMK_TorqueLimitPositivROP : RelationalOperator  Operator=<  OutDataTypeStr=boolean  RndMeth=Nearest
  AMK_TorqueLimitPositivRon : Rounding  Operator=round
  AMK_TorqueLimitPositivSW : Switch  Criteria=u2 ~= 0
  AMK_TorqueLimitPositiv_1sat : Saturate  UpperLimit=65535  LowerLimit=0
  AMK_TorqueLimitPositiv_And : simulink/Logic and Bit Operations/Bitwise Operator  logicop=AND  UseBitMask=off  NumInputPorts=2  BitMask=bin2dec('11011001')  BitMaskRealWorld=Stored Integer
  AMK_TorqueLimitPositiv_And_C : Constant  Value=255  OutDataTypeStr=uint32
  AMK_TorqueLimitPositiv_Convert : DataTypeConversion  OutDataTypeStr=uint32
  AMK_TorqueLimitPositiv_D : Product  Inputs=*/
  AMK_TorqueLimitPositiv_D1 : Product  Inputs=*/
  AMK_TorqueLimitPositiv_F : Constant  Value=0.1  OutDataTypeStr=single
  AMK_TorqueLimitPositiv_L : simulink/Logic and Bit Operations/Bitwise Operator  logicop=AND  UseBitMask=on  BitMask=65535  BitMaskRealWorld=Stored Integer
  AMK_TorqueLimitPositiv_O : Constant  Value=0  OutDataTypeStr=single
  AMK_TorqueLimitPositiv_S : ArithShift
  AMK_TorqueLimitPositiv_sat : Saturate  UpperLimit=100  LowerLimit=0
  AMK_TorqueLimitPositiv_st : Sum  Inputs=+-
  AMK_TorqueLimitPositivoutput6_C : Constant  Value=256
  AMK_TorqueLimitPositivsubcon : Sum  Inputs=+-
  BitCov : DataTypeConversion  OutDataTypeStr=uint8
  Constant{1..4,7..8} (6 alike) : Constant  Value=0  OutDataTypeStr=uint8  SampleTime=-1
  output1 : Outport
  output2 : Outport  Port=2
  output3 : Outport  Port=3
  output4 : Outport  Port=4
  output5 : Outport  Port=5
  output6 : Outport  Port=6
  output7 : Outport  Port=7
  output8 : Outport  Port=8
  wires:
  AMK_TorqueLimitPositiv/1 -> AMK_TorqueLimitPositiv_sat/1
  AMK_TorqueLimitPositiv_sat/1 -> AMK_TorqueLimitPositiv_st/1
  AMK_TorqueLimitPositiv_O/1 -> AMK_TorqueLimitPositiv_st/2
  AMK_TorqueLimitPositiv_st/1 -> AMK_TorqueLimitPositiv_D/1
  AMK_TorqueLimitPositiv_F/1 -> AMK_TorqueLimitPositiv_D/2
  AMK_TorqueLimitPositiv_D/1 -> AMK_TorqueLimitPositivRon/1
  AMK_TorqueLimitPositivRon/1 -> AMK_TorqueLimitPositivROP/1, AMK_TorqueLimitPositivABS/1, AMK_TorqueLimitPositivSW/3
  AMK_TorqueLimitPositivCosR/1 -> AMK_TorqueLimitPositivROP/2
  AMK_TorqueLimitPositivConS/1 -> AMK_TorqueLimitPositivCS/1
  AMK_TorqueLimitPositivCS/1 -> AMK_TorqueLimitPositivsubcon/1
  AMK_TorqueLimitPositivABS/1 -> AMK_TorqueLimitPositivsubcon/2
  AMK_TorqueLimitPositivsubcon/1 -> AMK_TorqueLimitPositivSW/1
  AMK_TorqueLimitPositivROP/1 -> AMK_TorqueLimitPositivSW/2
  AMK_TorqueLimitPositivSW/1 -> AMK_TorqueLimitPositiv_S/1
  AMK_TorqueLimitPositiv_S/1 -> AMK_TorqueLimitPositiv_1sat/1
  AMK_TorqueLimitPositiv_1sat/1 -> AMK_TorqueLimitPositiv_Convert/1
  AMK_TorqueLimitPositiv_Convert/1 -> AMK_TorqueLimitPositiv_L/1
  AMK_TorqueLimitPositiv_L/1 -> AMK_TorqueLimitPositiv_D1/1, AMK_TorqueLimitPositiv_And/1
  AMK_TorqueLimitPositivoutput6_C/1 -> AMK_TorqueLimitPositiv_D1/2
  AMK_TorqueLimitPositiv_D1/1 -> AMK_TorqueLimitPositivCOV/1
  AMK_TorqueLimitPositivCOV/1 -> output6/1
  AMK_TorqueLimitPositiv_And_C/1 -> AMK_TorqueLimitPositiv_And/2
  AMK_TorqueLimitPositiv_And/1 -> BitCov/1
  BitCov/1 -> output5/1
  Constant1/1 -> output1/1
  Constant2/1 -> output2/1
  Constant3/1 -> output3/1
  Constant4/1 -> output4/1
  Constant7/1 -> output7/1
  Constant8/1 -> output8/1

== system E55_1030/Function-Call Subsystem2/Triggered Subsystem/AMK_Setpoints_Motor2/AMK_Control ==
  AMK_Control : Inport
  AMK_ControlCOV : DataTypeConversion  OutDataTypeStr=uint8
  AMK_ControlRon : Rounding  Operator=round
  AMK_Control_1sat : Saturate  UpperLimit=65535  LowerLimit=0
  AMK_Control_And : simulink/Logic and Bit Operations/Bitwise Operator  logicop=AND  UseBitMask=off  NumInputPorts=2  BitMask=bin2dec('11011001')  BitMaskRealWorld=Stored Integer
  AMK_Control_And_C : Constant  Value=255  OutDataTypeStr=uint32
  AMK_Control_Convert : DataTypeConversion  OutDataTypeStr=uint32
  AMK_Control_D : Product  Inputs=*/
  AMK_Control_D1 : Product  Inputs=*/
  AMK_Control_F : Constant  OutDataTypeStr=single
  AMK_Control_L : simulink/Logic and Bit Operations/Bitwise Operator  logicop=AND  UseBitMask=on  BitMask=65535  BitMaskRealWorld=Stored Integer
  AMK_Control_O : Constant  Value=0  OutDataTypeStr=single
  AMK_Control_S : ArithShift
  AMK_Control_sat : Saturate  UpperLimit=65535  LowerLimit=0
  AMK_Control_st : Sum  Inputs=+-
  AMK_Controloutput2_C : Constant  Value=256
  BitCov : DataTypeConversion  OutDataTypeStr=uint8
  Constant{3..8} (6 alike) : Constant  Value=0  OutDataTypeStr=uint8  SampleTime=-1
  output1 : Outport
  output2 : Outport  Port=2
  output3 : Outport  Port=3
  output4 : Outport  Port=4
  output5 : Outport  Port=5
  output6 : Outport  Port=6
  output7 : Outport  Port=7
  output8 : Outport  Port=8
  wires:
  Constant8/1 -> output8/1
  Constant7/1 -> output7/1
  Constant6/1 -> output6/1
  Constant5/1 -> output5/1
  Constant4/1 -> output4/1
  Constant3/1 -> output3/1
  BitCov/1 -> output1/1
  AMK_Control_And/1 -> BitCov/1
  AMK_Control_And_C/1 -> AMK_Control_And/2
  AMK_ControlCOV/1 -> output2/1
  AMK_Control_D1/1 -> AMK_ControlCOV/1
  AMK_Controloutput2_C/1 -> AMK_Control_D1/2
  AMK_Control_L/1 -> AMK_Control_And/1, AMK_Control_D1/1
  AMK_Control_Convert/1 -> AMK_Control_L/1
  AMK_Control_1sat/1 -> AMK_Control_Convert/1
  AMK_Control_S/1 -> AMK_Control_1sat/1
  AMK_ControlRon/1 -> AMK_Control_S/1
  AMK_Control_D/1 -> AMK_ControlRon/1
  AMK_Control_F/1 -> AMK_Control_D/2
  AMK_Control_st/1 -> AMK_Control_D/1
  AMK_Control_O/1 -> AMK_Control_st/2
  AMK_Control_sat/1 -> AMK_Control_st/1
  AMK_Control/1 -> AMK_Control_sat/1

== system E55_1030/Function-Call Subsystem2/Triggered Subsystem/AMK_Setpoints_Motor2/AMK_TargetVelocity ==
  AMK_TargetVelocity : Inport
  AMK_TargetVelocityABS : Abs
  AMK_TargetVelocityCOV : DataTypeConversion  OutDataTypeStr=uint8
  AMK_TargetVelocityCS : ArithShift  BitShiftNumber=-16
  AMK_TargetVelocityConS : Constant  OutDataTypeStr=single
  AMK_TargetVelocityCosR : Constant  Value=0  OutDataTypeStr=uint8
  AMK_TargetVelocityROP : RelationalOperator  Operator=<  OutDataTypeStr=boolean  RndMeth=Nearest
  AMK_TargetVelocityRon : Rounding  Operator=round
  AMK_TargetVelocitySW : Switch  Criteria=u2 ~= 0
  AMK_TargetVelocity_1sat : Saturate  UpperLimit=65535  LowerLimit=0
  AMK_TargetVelocity_And : simulink/Logic and Bit Operations/Bitwise Operator  logicop=AND  UseBitMask=off  NumInputPorts=2  BitMask=bin2dec('11011001')  BitMaskRealWorld=Stored Integer
  AMK_TargetVelocity_And_C : Constant  Value=255  OutDataTypeStr=uint32
  AMK_TargetVelocity_Convert : DataTypeConversion  OutDataTypeStr=uint32
  AMK_TargetVelocity_D : Product  Inputs=*/
  AMK_TargetVelocity_D1 : Product  Inputs=*/
  AMK_TargetVelocity_F : Constant  OutDataTypeStr=single
  AMK_TargetVelocity_L : simulink/Logic and Bit Operations/Bitwise Operator  logicop=AND  UseBitMask=on  BitMask=65535  BitMaskRealWorld=Stored Integer
  AMK_TargetVelocity_O : Constant  Value=0  OutDataTypeStr=single
  AMK_TargetVelocity_S : ArithShift
  AMK_TargetVelocity_sat : Saturate  UpperLimit=32767  LowerLimit=-32768
  AMK_TargetVelocity_st : Sum  Inputs=+-
  AMK_TargetVelocityoutput4_C : Constant  Value=256
  AMK_TargetVelocitysubcon : Sum  Inputs=+-
  BitCov : DataTypeConversion  OutDataTypeStr=uint8
  Constant{1..2,5..8} (6 alike) : Constant  Value=0  OutDataTypeStr=uint8  SampleTime=-1
  output1 : Outport
  output2 : Outport  Port=2
  output3 : Outport  Port=3
  output4 : Outport  Port=4
  output5 : Outport  Port=5
  output6 : Outport  Port=6
  output7 : Outport  Port=7
  output8 : Outport  Port=8
  wires:
  Constant8/1 -> output8/1
  Constant7/1 -> output7/1
  Constant6/1 -> output6/1
  Constant5/1 -> output5/1
  Constant2/1 -> output2/1
  Constant1/1 -> output1/1
  BitCov/1 -> output3/1
  AMK_TargetVelocity_And/1 -> BitCov/1
  AMK_TargetVelocity_And_C/1 -> AMK_TargetVelocity_And/2
  AMK_TargetVelocityCOV/1 -> output4/1
  AMK_TargetVelocity_D1/1 -> AMK_TargetVelocityCOV/1
  AMK_TargetVelocityoutput4_C/1 -> AMK_TargetVelocity_D1/2
  AMK_TargetVelocity_L/1 -> AMK_TargetVelocity_And/1, AMK_TargetVelocity_D1/1
  AMK_TargetVelocity_Convert/1 -> AMK_TargetVelocity_L/1
  AMK_TargetVelocity_1sat/1 -> AMK_TargetVelocity_Convert/1
  AMK_TargetVelocity_S/1 -> AMK_TargetVelocity_1sat/1
  AMK_TargetVelocitySW/1 -> AMK_TargetVelocity_S/1
  AMK_TargetVelocityROP/1 -> AMK_TargetVelocitySW/2
  AMK_TargetVelocitysubcon/1 -> AMK_TargetVelocitySW/1
  AMK_TargetVelocityABS/1 -> AMK_TargetVelocitysubcon/2
  AMK_TargetVelocityCS/1 -> AMK_TargetVelocitysubcon/1
  AMK_TargetVelocityConS/1 -> AMK_TargetVelocityCS/1
  AMK_TargetVelocityCosR/1 -> AMK_TargetVelocityROP/2
  AMK_TargetVelocityRon/1 -> AMK_TargetVelocitySW/3, AMK_TargetVelocityABS/1, AMK_TargetVelocityROP/1
  AMK_TargetVelocity_D/1 -> AMK_TargetVelocityRon/1
  AMK_TargetVelocity_F/1 -> AMK_TargetVelocity_D/2
  AMK_TargetVelocity_st/1 -> AMK_TargetVelocity_D/1
  AMK_TargetVelocity_O/1 -> AMK_TargetVelocity_st/2
  AMK_TargetVelocity_sat/1 -> AMK_TargetVelocity_st/1
  AMK_TargetVelocity/1 -> AMK_TargetVelocity_sat/1

== system E55_1030/Function-Call Subsystem2/Triggered Subsystem/AMK_Setpoints_Motor2/AMK_TorqueLimitNegativ ==
  AMK_TorqueLimitNegativ : Inport
  AMK_TorqueLimitNegativABS : Abs
  AMK_TorqueLimitNegativCOV : DataTypeConversion  OutDataTypeStr=uint8
  AMK_TorqueLimitNegativCS : ArithShift  BitShiftNumber=-16
  AMK_TorqueLimitNegativConS : Constant  OutDataTypeStr=single
  AMK_TorqueLimitNegativCosR : Constant  Value=0  OutDataTypeStr=uint8
  AMK_TorqueLimitNegativROP : RelationalOperator  Operator=<  OutDataTypeStr=boolean  RndMeth=Nearest
  AMK_TorqueLimitNegativRon : Rounding  Operator=round
  AMK_TorqueLimitNegativSW : Switch  Criteria=u2 ~= 0
  AMK_TorqueLimitNegativ_1sat : Saturate  UpperLimit=65535  LowerLimit=0
  AMK_TorqueLimitNegativ_And : simulink/Logic and Bit Operations/Bitwise Operator  logicop=AND  UseBitMask=off  NumInputPorts=2  BitMask=bin2dec('11011001')  BitMaskRealWorld=Stored Integer
  AMK_TorqueLimitNegativ_And_C : Constant  Value=255  OutDataTypeStr=uint32
  AMK_TorqueLimitNegativ_Convert : DataTypeConversion  OutDataTypeStr=uint32
  AMK_TorqueLimitNegativ_D : Product  Inputs=*/
  AMK_TorqueLimitNegativ_D1 : Product  Inputs=*/
  AMK_TorqueLimitNegativ_F : Constant  Value=0.1  OutDataTypeStr=single
  AMK_TorqueLimitNegativ_L : simulink/Logic and Bit Operations/Bitwise Operator  logicop=AND  UseBitMask=on  BitMask=65535  BitMaskRealWorld=Stored Integer
  AMK_TorqueLimitNegativ_O : Constant  Value=0  OutDataTypeStr=single
  AMK_TorqueLimitNegativ_S : ArithShift
  AMK_TorqueLimitNegativ_sat : Saturate  UpperLimit=0  LowerLimit=-100
  AMK_TorqueLimitNegativ_st : Sum  Inputs=+-
  AMK_TorqueLimitNegativoutput8_C : Constant  Value=256
  AMK_TorqueLimitNegativsubcon : Sum  Inputs=+-
  BitCov : DataTypeConversion  OutDataTypeStr=uint8
  Constant{1..6} (6 alike) : Constant  Value=0  OutDataTypeStr=uint8  SampleTime=-1
  output1 : Outport
  output2 : Outport  Port=2
  output3 : Outport  Port=3
  output4 : Outport  Port=4
  output5 : Outport  Port=5
  output6 : Outport  Port=6
  output7 : Outport  Port=7
  output8 : Outport  Port=8
  wires:
  Constant6/1 -> output6/1
  Constant5/1 -> output5/1
  Constant4/1 -> output4/1
  Constant3/1 -> output3/1
  Constant2/1 -> output2/1
  Constant1/1 -> output1/1
  BitCov/1 -> output7/1
  AMK_TorqueLimitNegativ_And/1 -> BitCov/1
  AMK_TorqueLimitNegativ_And_C/1 -> AMK_TorqueLimitNegativ_And/2
  AMK_TorqueLimitNegativCOV/1 -> output8/1
  AMK_TorqueLimitNegativ_D1/1 -> AMK_TorqueLimitNegativCOV/1
  AMK_TorqueLimitNegativoutput8_C/1 -> AMK_TorqueLimitNegativ_D1/2
  AMK_TorqueLimitNegativ_L/1 -> AMK_TorqueLimitNegativ_And/1, AMK_TorqueLimitNegativ_D1/1
  AMK_TorqueLimitNegativ_Convert/1 -> AMK_TorqueLimitNegativ_L/1
  AMK_TorqueLimitNegativ_1sat/1 -> AMK_TorqueLimitNegativ_Convert/1
  AMK_TorqueLimitNegativ_S/1 -> AMK_TorqueLimitNegativ_1sat/1
  AMK_TorqueLimitNegativSW/1 -> AMK_TorqueLimitNegativ_S/1
  AMK_TorqueLimitNegativROP/1 -> AMK_TorqueLimitNegativSW/2
  AMK_TorqueLimitNegativsubcon/1 -> AMK_TorqueLimitNegativSW/1
  AMK_TorqueLimitNegativABS/1 -> AMK_TorqueLimitNegativsubcon/2
  AMK_TorqueLimitNegativCS/1 -> AMK_TorqueLimitNegativsubcon/1
  AMK_TorqueLimitNegativConS/1 -> AMK_TorqueLimitNegativCS/1
  AMK_TorqueLimitNegativCosR/1 -> AMK_TorqueLimitNegativROP/2
  AMK_TorqueLimitNegativRon/1 -> AMK_TorqueLimitNegativSW/3, AMK_TorqueLimitNegativABS/1, AMK_TorqueLimitNegativROP/1
  AMK_TorqueLimitNegativ_D/1 -> AMK_TorqueLimitNegativRon/1
  AMK_TorqueLimitNegativ_F/1 -> AMK_TorqueLimitNegativ_D/2
  AMK_TorqueLimitNegativ_st/1 -> AMK_TorqueLimitNegativ_D/1
  AMK_TorqueLimitNegativ_O/1 -> AMK_TorqueLimitNegativ_st/2
  AMK_TorqueLimitNegativ_sat/1 -> AMK_TorqueLimitNegativ_st/1
  AMK_TorqueLimitNegativ/1 -> AMK_TorqueLimitNegativ_sat/1

== system E55_1030/Function-Call Subsystem2/Triggered Subsystem/AMK_Setpoints_Motor2/AMK_TorqueLimitPositiv ==
  AMK_TorqueLimitPositiv : Inport
  AMK_TorqueLimitPositivABS : Abs
  AMK_TorqueLimitPositivCOV : DataTypeConversion  OutDataTypeStr=uint8
  AMK_TorqueLimitPositivCS : ArithShift  BitShiftNumber=-16
  AMK_TorqueLimitPositivConS : Constant  OutDataTypeStr=single
  AMK_TorqueLimitPositivCosR : Constant  Value=0  OutDataTypeStr=uint8
  AMK_TorqueLimitPositivROP : RelationalOperator  Operator=<  OutDataTypeStr=boolean  RndMeth=Nearest
  AMK_TorqueLimitPositivRon : Rounding  Operator=round
  AMK_TorqueLimitPositivSW : Switch  Criteria=u2 ~= 0
  AMK_TorqueLimitPositiv_1sat : Saturate  UpperLimit=65535  LowerLimit=0
  AMK_TorqueLimitPositiv_And : simulink/Logic and Bit Operations/Bitwise Operator  logicop=AND  UseBitMask=off  NumInputPorts=2  BitMask=bin2dec('11011001')  BitMaskRealWorld=Stored Integer
  AMK_TorqueLimitPositiv_And_C : Constant  Value=255  OutDataTypeStr=uint32
  AMK_TorqueLimitPositiv_Convert : DataTypeConversion  OutDataTypeStr=uint32
  AMK_TorqueLimitPositiv_D : Product  Inputs=*/
  AMK_TorqueLimitPositiv_D1 : Product  Inputs=*/
  AMK_TorqueLimitPositiv_F : Constant  Value=0.1  OutDataTypeStr=single
  AMK_TorqueLimitPositiv_L : simulink/Logic and Bit Operations/Bitwise Operator  logicop=AND  UseBitMask=on  BitMask=65535  BitMaskRealWorld=Stored Integer
  AMK_TorqueLimitPositiv_O : Constant  Value=0  OutDataTypeStr=single
  AMK_TorqueLimitPositiv_S : ArithShift
  AMK_TorqueLimitPositiv_sat : Saturate  UpperLimit=100  LowerLimit=0
  AMK_TorqueLimitPositiv_st : Sum  Inputs=+-
  AMK_TorqueLimitPositivoutput6_C : Constant  Value=256
  AMK_TorqueLimitPositivsubcon : Sum  Inputs=+-
  BitCov : DataTypeConversion  OutDataTypeStr=uint8
  Constant{1..4,7..8} (6 alike) : Constant  Value=0  OutDataTypeStr=uint8  SampleTime=-1
  output1 : Outport
  output2 : Outport  Port=2
  output3 : Outport  Port=3
  output4 : Outport  Port=4
  output5 : Outport  Port=5
  output6 : Outport  Port=6
  output7 : Outport  Port=7
  output8 : Outport  Port=8
  wires:
  Constant8/1 -> output8/1
  Constant7/1 -> output7/1
  Constant4/1 -> output4/1
  Constant3/1 -> output3/1
  Constant2/1 -> output2/1
  Constant1/1 -> output1/1
  BitCov/1 -> output5/1
  AMK_TorqueLimitPositiv_And/1 -> BitCov/1
  AMK_TorqueLimitPositiv_And_C/1 -> AMK_TorqueLimitPositiv_And/2
  AMK_TorqueLimitPositivCOV/1 -> output6/1
  AMK_TorqueLimitPositiv_D1/1 -> AMK_TorqueLimitPositivCOV/1
  AMK_TorqueLimitPositivoutput6_C/1 -> AMK_TorqueLimitPositiv_D1/2
  AMK_TorqueLimitPositiv_L/1 -> AMK_TorqueLimitPositiv_And/1, AMK_TorqueLimitPositiv_D1/1
  AMK_TorqueLimitPositiv_Convert/1 -> AMK_TorqueLimitPositiv_L/1
  AMK_TorqueLimitPositiv_1sat/1 -> AMK_TorqueLimitPositiv_Convert/1
  AMK_TorqueLimitPositiv_S/1 -> AMK_TorqueLimitPositiv_1sat/1
  AMK_TorqueLimitPositivSW/1 -> AMK_TorqueLimitPositiv_S/1
  AMK_TorqueLimitPositivROP/1 -> AMK_TorqueLimitPositivSW/2
  AMK_TorqueLimitPositivsubcon/1 -> AMK_TorqueLimitPositivSW/1
  AMK_TorqueLimitPositivABS/1 -> AMK_TorqueLimitPositivsubcon/2
  AMK_TorqueLimitPositivCS/1 -> AMK_TorqueLimitPositivsubcon/1
  AMK_TorqueLimitPositivConS/1 -> AMK_TorqueLimitPositivCS/1
  AMK_TorqueLimitPositivCosR/1 -> AMK_TorqueLimitPositivROP/2
  AMK_TorqueLimitPositivRon/1 -> AMK_TorqueLimitPositivSW/3, AMK_TorqueLimitPositivABS/1, AMK_TorqueLimitPositivROP/1
  AMK_TorqueLimitPositiv_D/1 -> AMK_TorqueLimitPositivRon/1
  AMK_TorqueLimitPositiv_F/1 -> AMK_TorqueLimitPositiv_D/2
  AMK_TorqueLimitPositiv_st/1 -> AMK_TorqueLimitPositiv_D/1
  AMK_TorqueLimitPositiv_O/1 -> AMK_TorqueLimitPositiv_st/2
  AMK_TorqueLimitPositiv_sat/1 -> AMK_TorqueLimitPositiv_st/1
  AMK_TorqueLimitPositiv/1 -> AMK_TorqueLimitPositiv_sat/1

== system E55_1030/Function-Call Subsystem2/Triggered Subsystem/AMK_Setpoints_Motor3/AMK_Control ==
  AMK_Control : Inport
  AMK_ControlCOV : DataTypeConversion  OutDataTypeStr=uint8
  AMK_ControlRon : Rounding  Operator=round
  AMK_Control_1sat : Saturate  UpperLimit=65535  LowerLimit=0
  AMK_Control_And : simulink/Logic and Bit Operations/Bitwise Operator  logicop=AND  UseBitMask=off  NumInputPorts=2  BitMask=bin2dec('11011001')  BitMaskRealWorld=Stored Integer
  AMK_Control_And_C : Constant  Value=255  OutDataTypeStr=uint32
  AMK_Control_Convert : DataTypeConversion  OutDataTypeStr=uint32
  AMK_Control_D : Product  Inputs=*/
  AMK_Control_D1 : Product  Inputs=*/
  AMK_Control_F : Constant  OutDataTypeStr=single
  AMK_Control_L : simulink/Logic and Bit Operations/Bitwise Operator  logicop=AND  UseBitMask=on  BitMask=65535  BitMaskRealWorld=Stored Integer
  AMK_Control_O : Constant  Value=0  OutDataTypeStr=single
  AMK_Control_S : ArithShift
  AMK_Control_sat : Saturate  UpperLimit=65535  LowerLimit=0
  AMK_Control_st : Sum  Inputs=+-
  AMK_Controloutput2_C : Constant  Value=256
  BitCov : DataTypeConversion  OutDataTypeStr=uint8
  Constant{3..8} (6 alike) : Constant  Value=0  OutDataTypeStr=uint8  SampleTime=-1
  output1 : Outport
  output2 : Outport  Port=2
  output3 : Outport  Port=3
  output4 : Outport  Port=4
  output5 : Outport  Port=5
  output6 : Outport  Port=6
  output7 : Outport  Port=7
  output8 : Outport  Port=8
  wires:
  Constant8/1 -> output8/1
  Constant7/1 -> output7/1
  Constant6/1 -> output6/1
  Constant5/1 -> output5/1
  Constant4/1 -> output4/1
  Constant3/1 -> output3/1
  BitCov/1 -> output1/1
  AMK_Control_And/1 -> BitCov/1
  AMK_Control_And_C/1 -> AMK_Control_And/2
  AMK_ControlCOV/1 -> output2/1
  AMK_Control_D1/1 -> AMK_ControlCOV/1
  AMK_Controloutput2_C/1 -> AMK_Control_D1/2
  AMK_Control_L/1 -> AMK_Control_And/1, AMK_Control_D1/1
  AMK_Control_Convert/1 -> AMK_Control_L/1
  AMK_Control_1sat/1 -> AMK_Control_Convert/1
  AMK_Control_S/1 -> AMK_Control_1sat/1
  AMK_ControlRon/1 -> AMK_Control_S/1
  AMK_Control_D/1 -> AMK_ControlRon/1
  AMK_Control_F/1 -> AMK_Control_D/2
  AMK_Control_st/1 -> AMK_Control_D/1
  AMK_Control_O/1 -> AMK_Control_st/2
  AMK_Control_sat/1 -> AMK_Control_st/1
  AMK_Control/1 -> AMK_Control_sat/1

== system E55_1030/Function-Call Subsystem2/Triggered Subsystem/AMK_Setpoints_Motor3/AMK_TargetVelocity ==
  AMK_TargetVelocity : Inport
  AMK_TargetVelocityABS : Abs
  AMK_TargetVelocityCOV : DataTypeConversion  OutDataTypeStr=uint8
  AMK_TargetVelocityCS : ArithShift  BitShiftNumber=-16
  AMK_TargetVelocityConS : Constant  OutDataTypeStr=single
  AMK_TargetVelocityCosR : Constant  Value=0  OutDataTypeStr=uint8
  AMK_TargetVelocityROP : RelationalOperator  Operator=<  OutDataTypeStr=boolean  RndMeth=Nearest
  AMK_TargetVelocityRon : Rounding  Operator=round
  AMK_TargetVelocitySW : Switch  Criteria=u2 ~= 0
  AMK_TargetVelocity_1sat : Saturate  UpperLimit=65535  LowerLimit=0
  AMK_TargetVelocity_And : simulink/Logic and Bit Operations/Bitwise Operator  logicop=AND  UseBitMask=off  NumInputPorts=2  BitMask=bin2dec('11011001')  BitMaskRealWorld=Stored Integer
  AMK_TargetVelocity_And_C : Constant  Value=255  OutDataTypeStr=uint32
  AMK_TargetVelocity_Convert : DataTypeConversion  OutDataTypeStr=uint32
  AMK_TargetVelocity_D : Product  Inputs=*/
  AMK_TargetVelocity_D1 : Product  Inputs=*/
  AMK_TargetVelocity_F : Constant  OutDataTypeStr=single
  AMK_TargetVelocity_L : simulink/Logic and Bit Operations/Bitwise Operator  logicop=AND  UseBitMask=on  BitMask=65535  BitMaskRealWorld=Stored Integer
  AMK_TargetVelocity_O : Constant  Value=0  OutDataTypeStr=single
  AMK_TargetVelocity_S : ArithShift
  AMK_TargetVelocity_sat : Saturate  UpperLimit=32767  LowerLimit=-32768
  AMK_TargetVelocity_st : Sum  Inputs=+-
  AMK_TargetVelocityoutput4_C : Constant  Value=256
  AMK_TargetVelocitysubcon : Sum  Inputs=+-
  BitCov : DataTypeConversion  OutDataTypeStr=uint8
  Constant{1..2,5..8} (6 alike) : Constant  Value=0  OutDataTypeStr=uint8  SampleTime=-1
  output1 : Outport
  output2 : Outport  Port=2
  output3 : Outport  Port=3
  output4 : Outport  Port=4
  output5 : Outport  Port=5
  output6 : Outport  Port=6
  output7 : Outport  Port=7
  output8 : Outport  Port=8
  wires:
  Constant8/1 -> output8/1
  Constant7/1 -> output7/1
  Constant6/1 -> output6/1
  Constant5/1 -> output5/1
  Constant2/1 -> output2/1
  Constant1/1 -> output1/1
  BitCov/1 -> output3/1
  AMK_TargetVelocity_And/1 -> BitCov/1
  AMK_TargetVelocity_And_C/1 -> AMK_TargetVelocity_And/2
  AMK_TargetVelocityCOV/1 -> output4/1
  AMK_TargetVelocity_D1/1 -> AMK_TargetVelocityCOV/1
  AMK_TargetVelocityoutput4_C/1 -> AMK_TargetVelocity_D1/2
  AMK_TargetVelocity_L/1 -> AMK_TargetVelocity_And/1, AMK_TargetVelocity_D1/1
  AMK_TargetVelocity_Convert/1 -> AMK_TargetVelocity_L/1
  AMK_TargetVelocity_1sat/1 -> AMK_TargetVelocity_Convert/1
  AMK_TargetVelocity_S/1 -> AMK_TargetVelocity_1sat/1
  AMK_TargetVelocitySW/1 -> AMK_TargetVelocity_S/1
  AMK_TargetVelocityROP/1 -> AMK_TargetVelocitySW/2
  AMK_TargetVelocitysubcon/1 -> AMK_TargetVelocitySW/1
  AMK_TargetVelocityABS/1 -> AMK_TargetVelocitysubcon/2
  AMK_TargetVelocityCS/1 -> AMK_TargetVelocitysubcon/1
  AMK_TargetVelocityConS/1 -> AMK_TargetVelocityCS/1
  AMK_TargetVelocityCosR/1 -> AMK_TargetVelocityROP/2
  AMK_TargetVelocityRon/1 -> AMK_TargetVelocitySW/3, AMK_TargetVelocityABS/1, AMK_TargetVelocityROP/1
  AMK_TargetVelocity_D/1 -> AMK_TargetVelocityRon/1
  AMK_TargetVelocity_F/1 -> AMK_TargetVelocity_D/2
  AMK_TargetVelocity_st/1 -> AMK_TargetVelocity_D/1
  AMK_TargetVelocity_O/1 -> AMK_TargetVelocity_st/2
  AMK_TargetVelocity_sat/1 -> AMK_TargetVelocity_st/1
  AMK_TargetVelocity/1 -> AMK_TargetVelocity_sat/1
